simulink model "rear_differencial_dense_1"  (R2022b)
settings: Solver=FixedStepDiscrete  StartTime=0.0  StopTime=10.0  FixedStep=0.001  RelTol=1e-3  EnableMultiTasking=on
PreLoadFcn:
  | PowerOn_data
InitFcn:
  | EcoCoder_PreCheckLic();
values from neighbouring files (symbols this model uses):
  Accelerate_Percent_BreakPoints = uint8([0  2  5  10  20  30  40  50  60  70  80  90  100])    [PowerOn_data.m]
  MotorSpeed_BreakPoints = uint16(linspace(0,18000,13))    [PowerOn_data.m]
  Torque_Table = int8([ ... (first row only)    [PowerOn_data.m]
undefined symbols (not defined in the file or in its folder): HV_Botton, Inverter_Button, SC_Closed
libraries: CoderSF_BSW_Libs x83, SF_CanService_Libs x17, CoderSF_ADC2Volt_Libs x5, simulink x2, dspswit3 x1
(part 1 of 2)
settings Model: Param_HCUVersion=EV22297A  Creator=hxf  LastModifiedBy=Woler
settings SolverCC: AlgebraicLoopSolver=TrustRegion
settings DataIOCC: SaveFormat=Structure  SignalLoggingSaveFormat=ModelDataLogs  SaveOutput=off  SignalLogging=off  DSMLogging=off  SaveTime=off  ReturnWorkspaceOutputs=off
settings OptimizationCC: DefaultParameterBehavior=Inlined  InlineInvariantSignals=on  EnhancedBackFolding=on  StrengthReduction=on  EnableMemcpy=off  PassReuseOutputArgsAs=Individual arguments  EfficientFloat2IntCast=on  LifeSpan=1  SimCompilerOptimization=on  OptimizeBlockOrder=speed  DifferentSizesBufferReuse=on  EfficientTunableParamExpr=on
settings DebuggingCC: AlgebraicLoopMsg=none  ArtificialAlgebraicLoopMsg=none  SaveWithDisabledLinksMsg=none  SaveWithParameterizedLinksMsg=none  CheckSSInitialOutputMsg=off  UnderspecifiedInitializationDetection=Classic  SignalResolutionControl=TryResolveAll  BlockPriorityViolationMsg=error  MinStepSizeMsg=none  InheritedTsInSrcMsg=none  MultiTaskDSMMsg=none  MultiTaskCondExecSysMsg=none  MultiTaskRateTransMsg=warning  TasksWithSamePriorityMsg=none  SigSpecEnsureSampleTimeMsg=none  IntegerOverflowMsg=error  Int32ToFloatConvMsg=none  ParameterPrecisionLossMsg=none  ParameterTunabilityLossMsg=none  FixptConstOverflowMsg=error  FcnCallInpInsideContextMsg=warning  UnconnectedInputMsg=error  UnconnectedOutputMsg=error  UnconnectedLineMsg=error  FrameProcessingCompatibilityMsg=none  BusObjectLabelMismatch=none  RootOutportRequireBusObject=none  UnknownTsInhSupMsg=none  ModelReferenceDataLoggingMessage=none  OperatingPointInterfaceChecksumMismatchMsg=none  SFUnusedDataAndEventsDiag=none  SFUnexpectedBacktrackingDiag=none  SFInvalidInputDataAccessInChartInitDiag=none  SFNoUnconditionalDefaultTransitionDiag=none  SFTransitionOutsideNaturalParentDiag=none  SFUnreachableExecutionPathDiag=none  SFMachineParentedDataDiag=warning  ArithmeticOperatorsInVariantConditions=warning
settings HardwareCC: ProdBitPerPointer=32  ProdBitPerSizeT=32  ProdBitPerPtrDiffT=32  ProdLargestAtomicFloat=None  ProdWordSize=32  ProdHWDeviceType=Infineon->TriCore
settings ModelReferenceCC: UpdateModelReferenceTargets=Force  EnableRefExpFcnMdlSchedulingChecks=on  ModelReferenceNumInstancesAllowed=Single  PropagateSignalLabelsOutOfModel=off
settings SFSimCC: SFSimEcho=off  MATLABDynamicMemAlloc=off  CustomCodeUndefinedFunction=UseInterfaceOnly
settings RTWCC: Description=Ecotrons TC27x  SystemTargetFile=EcoCoderTC27x.tlc  GenerateMakefile=off  TemplateMakefile=ert_default_tmf  RTWVerbose=off  RetainRTWFile=on  RTWCompilerOptimization=on
settings CodeAppCC: IgnoreCustomStorageClasses=off  OperatorAnnotations=on  CustomSymbolStrGlobalVar=$N$M  CustomSymbolStrType=$N$M  CustomSymbolStrFcn=$N$M  CustomSymbolStrFcnArg=$N$M  CustomSymbolStrBlkIO=$N$M  CustomSymbolStrMacro=$N$M
settings STFCustomTargetCC: UtilityFuncGeneration=Shared location  MultiwordLength=256  IncludeMdlTerminateFcn=off  CombineOutputUpdateFcns=on  SuppressErrorStatus=on  ERTCustomFileBanners=on  SupportComplex=off  SupportContinuousTime=off  SupportNonInlinedSFcns=off  MATLABClassNameForMDSCustomization=Simulink.SoftwareTarget.ERTCustomization  SystemTargetFile=EcoCoderTC27x.tlc
settings ERTTargetCC: UtilityFuncGeneration=Shared location  ParMdlRefBuildCompliant=off  CompOptLevelCompliant=off  ConcurrentExecutionCompliant=off  IncludeMdlTerminateFcn=off  SuppressErrorStatus=on  SupportComplex=off  RemoveResetFunc=off  ModelStepFunctionPrototypeControlCompliant=off  CPPClassGenCompliant=off  UseToolchainInfoCompliant=off  GenerateASAP2=on  InlinedParameterPlacement=NonHierarchical  ERTCustomFileTemplate=MPC5644A_file_process.tlc  ERTFilePackagingFormat=Compact  PreserveIfCondition=on  ConvertIfToSwitch=off  PreserveExternInFcnDecls=off  SuppressUnreachableDefaultCases=off

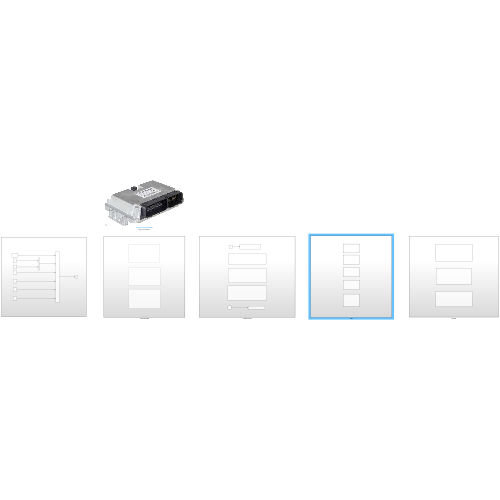
[thumbnail: Simulink's stored preview of the top-level diagram]
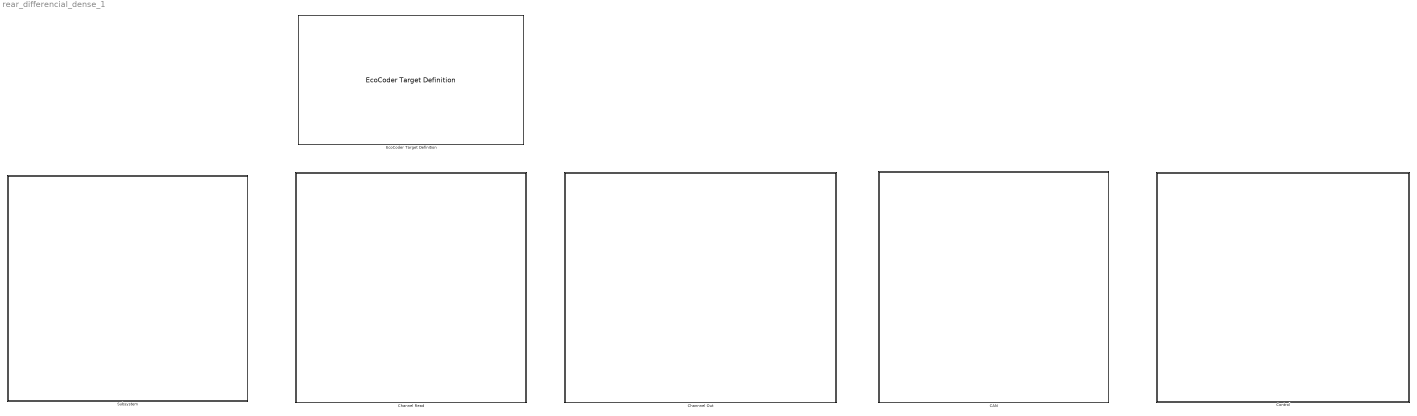
== system rear_differencial_dense_1 ==
  CAN : Subsystem
  Channel Read : Subsystem
  Channnel Out : Subsystem
  Control : Subsystem
  EcoCoder Target Definition : CoderSF_BSW_Libs/EcoCoder Target Definition  targetECU=EV22297A  EcoCoderBlockID=T001_Target  enNoTriggerCall=on  flgBlockReduction=on  flgShowDebugDisp=off  flgDisTargetOutFIleCounter=off  flgClearAllOldFiles=on  tc275_cal_len=hex2dec('00008000')  ipVal='192.168.0.123'  userName='nvidia'  passWord='nvidia'  workSpace='~/cmake_ws'  libraryLink=''  enExt=on  portExt=17725  internal_flash=[hex2dec('00020000'),hex2dec('000E0000')]  cal_rom_phy=[hex2dec('00010000'),hex2dec('00002000')]  cal_ram_wp=[hex2dec('4000F000'),hex2dec('00002000')]  cal_ram_msm=[hex2dec('40000000'),hex2dec('00002000')]  var_ram_wp=[hex2dec('40002000'),hex2dec('0000D000')]  write_back_fixed_ram=[hex2dec('40011000'),hex2dec('00001000')]  write_back_unfixed_ram=[hex2dec('40012000'),hex2dec('00001000')]  stack=[hex2dec('40013000'),hex2dec('00001000')]
      settings: AttributesFormatString=Target :%<targetECU>
  Subsystem : Subsystem

== system rear_differencial_dense_1/CAN ==
  CAN Definition : Subsystem
  CAN Read : Subsystem
  CAN Write : Subsystem
  Fixed CCP Slave Definition : CoderSF_BSW_Libs/CCP/Fixed CCP Slave Definition  ccp_enSet=on  ccp_disASW=off  channel=CAN_B  stationaddressSet=hex2dec('0112')  croidSet=hex2dec('200')  dtoidSet=hex2dec('201')  daqidSet=[hex2dec('210') hex2dec('211') hex2dec('212') hex2dec('213')]  daqpidSet=[hex2dec('0') hex2dec('0') hex2dec('0') hex2dec('0')]  daqlenSet=[hex2dec('A') hex2dec('20') hex2dec('30') hex2dec('50')]  daqperSet=[10 20 100 200]  EcoCoderBlockID=C002_CCP21Conf
  Write CAN Measurement : Subsystem

== system rear_differencial_dense_1/Channel Read ==
  ADC : Subsystem
  DI : Subsystem
  Multi_geer_knob : Subsystem

== system rear_differencial_dense_1/Channnel Out ==
  Constant : Constant  OutDataTypeStr=boolean
  Constant1 : Constant  OutDataTypeStr=boolean
  Power Control Output : CoderSF_BSW_Libs/System Management Blocks/Power Control Output  channel=PWR5V3
  Switch Output : CoderSF_BSW_Libs/Digital I//O/Switch Output  channel=HSO07
  水泵风扇 : Subsystem
  电池箱ACC_on : Subsystem
  蜂鸣器 : Subsystem
  wires:
  Constant1/1 -> Power Control Output/1
  Constant/1 -> Switch Output/1

== system rear_differencial_dense_1/Control ==
  Motor_Enable : Subsystem
  StateMachine : Subsystem
  Torque_Control : Subsystem

== system rear_differencial_dense_1/Subsystem ==
  Bus Creator : BusCreator  Inputs=Wheelbase,Distribution of Axle Load,Front Length,Rear Length,Front Track Width,Rear Track Width
  Divide : Product  Inputs=*/
  Front Length : Constant  Value=0.79
  Front Mass : Constant  Value=110
  Front Track Width : Constant  Value=1.2
  Rear Length : Constant  Value=0.79
  Rear Mass : Constant  Value=135
  Rear Track Width : Constant  Value=1.16
  Terminator : Terminator
  Wheelbase : Constant  Value=1.58
  wires:
  Front Mass/1 -> Divide/1
  Rear Mass/1 -> Divide/2
  Divide/1 -> Bus Creator/2  "Distribution of Axle Load"
  Wheelbase/1 -> Bus Creator/1  "Wheelbase"
  Front Length/1 -> Bus Creator/3  "Front Length"
  Rear Length/1 -> Bus Creator/4  "Rear Length"
  Front Track Width/1 -> Bus Creator/5  "Front Track Width"
  Rear Track Width/1 -> Bus Creator/6  "Rear Track Width"
  Bus Creator/1 -> Terminator/1

== system rear_differencial_dense_1/CAN/CAN Definition ==
  CAN Channel Definition : CoderSF_BSW_Libs/CAN/CAN Channel Definition  channel=CAN_A  can_en=on  can_idfilter=off  can_rxextended=off  can_rxMask=hex2dec('7ff')  can_rxID=hex2dec('100')  can_baudrateIndex=250  can_txbuffer_size=200  can_rxbuffer_size=1  can_en_fd=off  nominalSamplePoint=7500  can_baudrateIndex_data=500  fastSamplePoint=7500  canfd_txbuffer_size=5  EcoCoderBlockID=C001_CANDef
  CAN Channel Definition1 : CoderSF_BSW_Libs/CAN/CAN Channel Definition  channel=CAN_B  can_en=on  can_idfilter=off  can_rxextended=off  can_rxMask=hex2dec('7ff')  can_rxID=hex2dec('100')  can_baudrateIndex=500  can_txbuffer_size=200  can_rxbuffer_size=1  can_en_fd=off  nominalSamplePoint=7500  can_baudrateIndex_data=500  fastSamplePoint=7500  canfd_txbuffer_size=5  EcoCoderBlockID=C001_CANDef
  CAN Channel Definition2 : CoderSF_BSW_Libs/CAN/CAN Channel Definition  channel=CAN_C  can_en=on  can_idfilter=off  can_rxextended=off  can_rxMask=hex2dec('7ff')  can_rxID=hex2dec('100')  can_baudrateIndex=500  can_txbuffer_size=20  can_rxbuffer_size=1  can_en_fd=off  nominalSamplePoint=7500  can_baudrateIndex_data=500  fastSamplePoint=7500  canfd_txbuffer_size=5  EcoCoderBlockID=C001_CANDef
  CAN Channel Definition3 : CoderSF_BSW_Libs/CAN/CAN Channel Definition  channel=CAN_D  can_en=on  can_idfilter=off  can_rxextended=off  can_rxMask=hex2dec('7ff')  can_rxID=hex2dec('100')  can_baudrateIndex=500  can_txbuffer_size=20  can_rxbuffer_size=1  can_en_fd=off  nominalSamplePoint=7500  can_baudrateIndex_data=500  fastSamplePoint=7500  canfd_txbuffer_size=5  EcoCoderBlockID=C001_CANDef
  CAN Channel Definition4 : CoderSF_BSW_Libs/CAN/CAN Channel Definition  channel=CAN_E  can_en=on  can_idfilter=off  can_rxextended=off  can_rxMask=hex2dec('7ff')  can_rxID=hex2dec('100')  can_baudrateIndex=250  can_txbuffer_size=20  can_rxbuffer_size=1  can_en_fd=off  nominalSamplePoint=7500  can_baudrateIndex_data=500  fastSamplePoint=7500  canfd_txbuffer_size=5  EcoCoderBlockID=C001_CANDef

== system rear_differencial_dense_1/CAN/CAN Read ==
  BMS_CAN : Subsystem
  Motor_CAN : Subsystem
  SAS__CAN : Subsystem

== system rear_differencial_dense_1/CAN/CAN Write ==
  Send_To_Inverter : Subsystem
  Send_To_Recorder : Subsystem

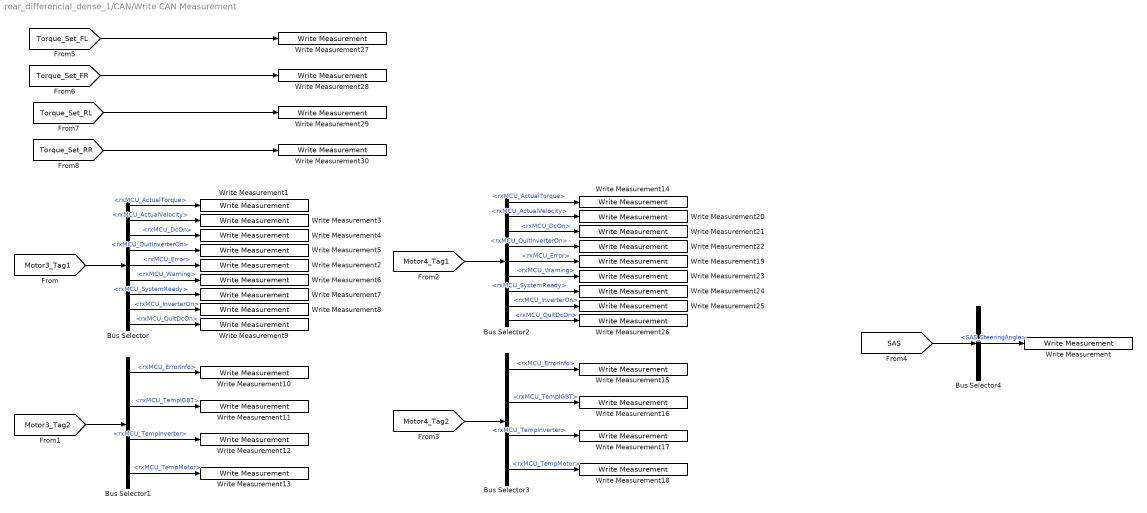
== system rear_differencial_dense_1/CAN/Write CAN Measurement ==
  Bus Selector : BusSelector  OutputSignals=rxMCU_ActualTorque,rxMCU_ActualVelocity,rxMCU_DcOn,rxMCU_QuitInverterOn,rxMCU_Error,rxMCU_Warning,rxMCU_SystemReady,rxMCU_InverterOn,rxMCU_QuitDcOn
  Bus Selector1 : BusSelector  OutputSignals=rxMCU_ErrorInfo,rxMCU_TempIGBT,rxMCU_TempInverter,rxMCU_TempMotor
  Bus Selector2 : BusSelector  OutputSignals=rxMCU_ActualTorque,rxMCU_ActualVelocity,rxMCU_DcOn,rxMCU_QuitInverterOn,rxMCU_Error,rxMCU_Warning,rxMCU_SystemReady,rxMCU_InverterOn,rxMCU_QuitDcOn
  Bus Selector3 : BusSelector  OutputSignals=rxMCU_ErrorInfo,rxMCU_TempIGBT,rxMCU_TempInverter,rxMCU_TempMotor
  Bus Selector4 : BusSelector  OutputSignals=SAS_SteeringAngle
  Write Measurement : CoderSF_BSW_Libs/Calibration & Measurement/Write Measurement  variable_name=Steering_Angle  variable_value=0  variable_type=single  numD=1  unitStr=""  descStr=""
      settings: AttributesFormatString=type:%<variable_type> Dimensions:%<numD>
  Write Measurement1 : CoderSF_BSW_Libs/Calibration & Measurement/Write Measurement  variable_name=RL_Actual_Torque  variable_value=0  variable_type=single  numD=1  unitStr=""  descStr=""
      settings: AttributesFormatString=type:%<variable_type> Dimensions:%<numD>
  Write Measurement10 : CoderSF_BSW_Libs/Calibration & Measurement/Write Measurement  variable_name=RL_Error_Info  variable_value=0  variable_type=uint16  numD=1  unitStr=""  descStr=""
      settings: AttributesFormatString=type:%<variable_type> Dimensions:%<numD>
  Write Measurement11 : CoderSF_BSW_Libs/Calibration & Measurement/Write Measurement  variable_name=RL_TempIGBT  variable_value=0  variable_type=single  numD=1  unitStr=""  descStr=""
      settings: AttributesFormatString=type:%<variable_type> Dimensions:%<numD>
  Write Measurement12 : CoderSF_BSW_Libs/Calibration & Measurement/Write Measurement  variable_name=RL_TempInverter  variable_value=0  variable_type=single  numD=1  unitStr=""  descStr=""
      settings: AttributesFormatString=type:%<variable_type> Dimensions:%<numD>
  Write Measurement13 : CoderSF_BSW_Libs/Calibration & Measurement/Write Measurement  variable_name=RL_TempMotor  variable_value=0  variable_type=single  numD=1  unitStr=""  descStr=""
      settings: AttributesFormatString=type:%<variable_type> Dimensions:%<numD>
  Write Measurement14 : CoderSF_BSW_Libs/Calibration & Measurement/Write Measurement  variable_name=RR_Actual_Torque  variable_value=0  variable_type=single  numD=1  unitStr=""  descStr=""
      settings: AttributesFormatString=type:%<variable_type> Dimensions:%<numD>
  Write Measurement15 : CoderSF_BSW_Libs/Calibration & Measurement/Write Measurement  variable_name=RR_Error_Info  variable_value=0  variable_type=uint16  numD=1  unitStr=""  descStr=""
      settings: AttributesFormatString=type:%<variable_type> Dimensions:%<numD>
  Write Measurement16 : CoderSF_BSW_Libs/Calibration & Measurement/Write Measurement  variable_name=RR_TempIGBT  variable_value=0  variable_type=single  numD=1  unitStr=""  descStr=""
      settings: AttributesFormatString=type:%<variable_type> Dimensions:%<numD>
  Write Measurement17 : CoderSF_BSW_Libs/Calibration & Measurement/Write Measurement  variable_name=RR_TempInverter  variable_value=0  variable_type=single  numD=1  unitStr=""  descStr=""
      settings: AttributesFormatString=type:%<variable_type> Dimensions:%<numD>
  Write Measurement18 : CoderSF_BSW_Libs/Calibration & Measurement/Write Measurement  variable_name=RR_TempMotor  variable_value=0  variable_type=single  numD=1  unitStr=""  descStr=""
      settings: AttributesFormatString=type:%<variable_type> Dimensions:%<numD>
  Write Measurement19 : CoderSF_BSW_Libs/Calibration & Measurement/Write Measurement  variable_name=RR_Error  variable_value=0  variable_type=boolean  numD=1  unitStr=""  descStr=""
      settings: AttributesFormatString=type:%<variable_type> Dimensions:%<numD>
  Write Measurement2 : CoderSF_BSW_Libs/Calibration & Measurement/Write Measurement  variable_name=RL_Error  variable_value=0  variable_type=boolean  numD=1  unitStr=""  descStr=""
      settings: AttributesFormatString=type:%<variable_type> Dimensions:%<numD>
  Write Measurement20 : CoderSF_BSW_Libs/Calibration & Measurement/Write Measurement  variable_name=RR_Actual_Velocity  variable_value=0  variable_type=int16  numD=1  unitStr=""  descStr=""
      settings: AttributesFormatString=type:%<variable_type> Dimensions:%<numD>
  Write Measurement21 : CoderSF_BSW_Libs/Calibration & Measurement/Write Measurement  variable_name=RR_DCon  variable_value=0  variable_type=boolean  numD=1  unitStr=""  descStr=""
      settings: AttributesFormatString=type:%<variable_type> Dimensions:%<numD>
  Write Measurement22 : CoderSF_BSW_Libs/Calibration & Measurement/Write Measurement  variable_name=RR_Quit_Inverter_on  variable_value=0  variable_type=boolean  numD=1  unitStr=""  descStr=""
      settings: AttributesFormatString=type:%<variable_type> Dimensions:%<numD>
  Write Measurement23 : CoderSF_BSW_Libs/Calibration & Measurement/Write Measurement  variable_name=RR_Warning  variable_value=0  variable_type=boolean  numD=1  unitStr=""  descStr=""
      settings: AttributesFormatString=type:%<variable_type> Dimensions:%<numD>
  Write Measurement24 : CoderSF_BSW_Libs/Calibration & Measurement/Write Measurement  variable_name=RR_System_Ready  variable_value=0  variable_type=boolean  numD=1  unitStr=""  descStr=""
      settings: AttributesFormatString=type:%<variable_type> Dimensions:%<numD>
  Write Measurement25 : CoderSF_BSW_Libs/Calibration & Measurement/Write Measurement  variable_name=RR_Inverter_on  variable_value=0  variable_type=boolean  numD=1  unitStr=""  descStr=""
      settings: AttributesFormatString=type:%<variable_type> Dimensions:%<numD>
  Write Measurement26 : CoderSF_BSW_Libs/Calibration & Measurement/Write Measurement  variable_name=RR_QuitDCon  variable_value=0  variable_type=boolean  numD=1  unitStr=""  descStr=""
      settings: AttributesFormatString=type:%<variable_type> Dimensions:%<numD>
  Write Measurement27 : CoderSF_BSW_Libs/Calibration & Measurement/Write Measurement  variable_name=Torque_Set_FL  variable_value=0  variable_type=uint16  numD=1  unitStr=""  descStr=""
      settings: AttributesFormatString=type:%<variable_type> Dimensions:%<numD>
  Write Measurement28 : CoderSF_BSW_Libs/Calibration & Measurement/Write Measurement  variable_name=Torque_Set_FR  variable_value=0  variable_type=uint16  numD=1  unitStr=""  descStr=""
      settings: AttributesFormatString=type:%<variable_type> Dimensions:%<numD>
  Write Measurement29 : CoderSF_BSW_Libs/Calibration & Measurement/Write Measurement  variable_name=Torque_Set_RL  variable_value=0  variable_type=uint16  numD=1  unitStr=""  descStr=""
      settings: AttributesFormatString=type:%<variable_type> Dimensions:%<numD>
  Write Measurement3 : CoderSF_BSW_Libs/Calibration & Measurement/Write Measurement  variable_name=RL_Actual_Velocity  variable_value=0  variable_type=int16  numD=1  unitStr=""  descStr=""
      settings: AttributesFormatString=type:%<variable_type> Dimensions:%<numD>
  Write Measurement30 : CoderSF_BSW_Libs/Calibration & Measurement/Write Measurement  variable_name=Torque_Set_RR  variable_value=0  variable_type=uint16  numD=1  unitStr=""  descStr=""
      settings: AttributesFormatString=type:%<variable_type> Dimensions:%<numD>
  Write Measurement4 : CoderSF_BSW_Libs/Calibration & Measurement/Write Measurement  variable_name=RL_DCon  variable_value=0  variable_type=boolean  numD=1  unitStr=""  descStr=""
      settings: AttributesFormatString=type:%<variable_type> Dimensions:%<numD>
  Write Measurement5 : CoderSF_BSW_Libs/Calibration & Measurement/Write Measurement  variable_name=RL_Quit_Inverter_on  variable_value=0  variable_type=boolean  numD=1  unitStr=""  descStr=""
      settings: AttributesFormatString=type:%<variable_type> Dimensions:%<numD>
  Write Measurement6 : CoderSF_BSW_Libs/Calibration & Measurement/Write Measurement  variable_name=RL_Warning  variable_value=0  variable_type=boolean  numD=1  unitStr=""  descStr=""
      settings: AttributesFormatString=type:%<variable_type> Dimensions:%<numD>
  Write Measurement7 : CoderSF_BSW_Libs/Calibration & Measurement/Write Measurement  variable_name=RL_System_Ready  variable_value=0  variable_type=boolean  numD=1  unitStr=""  descStr=""
      settings: AttributesFormatString=type:%<variable_type> Dimensions:%<numD>
  Write Measurement8 : CoderSF_BSW_Libs/Calibration & Measurement/Write Measurement  variable_name=RL_Inverter_on  variable_value=0  variable_type=boolean  numD=1  unitStr=""  descStr=""
      settings: AttributesFormatString=type:%<variable_type> Dimensions:%<numD>
  Write Measurement9 : CoderSF_BSW_Libs/Calibration & Measurement/Write Measurement  variable_name=RL_QuitDCon  variable_value=0  variable_type=boolean  numD=1  unitStr=""  descStr=""
      settings: AttributesFormatString=type:%<variable_type> Dimensions:%<numD>
  wires:
  Bus Selector1/4 -> Write Measurement13/1  "<rxMCU_TempMotor>"
  Bus Selector/1 -> Write Measurement1/1  "<rxMCU_ActualTorque>"
  Bus Selector2/9 -> Write Measurement26/1  "<rxMCU_QuitDcOn>"
  Bus Selector/2 -> Write Measurement3/1  "<rxMCU_ActualVelocity>"
  Bus Selector2/6 -> Write Measurement23/1  "<rxMCU_Warning>"
  Bus Selector/9 -> Write Measurement9/1  "<rxMCU_QuitDcOn>"
  Bus Selector/4 -> Write Measurement5/1  "<rxMCU_QuitInverterOn>"
  Bus Selector3/1 -> Write Measurement15/1  "<rxMCU_ErrorInfo>"
  Bus Selector3/3 -> Write Measurement17/1  "<rxMCU_TempInverter>"
  Bus Selector/3 -> Write Measurement4/1  "<rxMCU_DcOn>"
  [Motor3_Tag2] -> Bus Selector1/1
  Bus Selector/6 -> Write Measurement6/1  "<rxMCU_Warning>"
  Bus Selector/8 -> Write Measurement8/1  "<rxMCU_InverterOn>"
  Bus Selector/5 -> Write Measurement2/1  "<rxMCU_Error>"
  [Motor4_Tag2] -> Bus Selector3/1
  [Motor3_Tag1] -> Bus Selector/1
  Bus Selector2/2 -> Write Measurement20/1  "<rxMCU_ActualVelocity>"
  Bus Selector2/1 -> Write Measurement14/1  "<rxMCU_ActualTorque>"
  Bus Selector3/4 -> Write Measurement18/1  "<rxMCU_TempMotor>"
  Bus Selector2/5 -> Write Measurement19/1  "<rxMCU_Error>"
  Bus Selector2/8 -> Write Measurement25/1  "<rxMCU_InverterOn>"
  Bus Selector3/2 -> Write Measurement16/1  "<rxMCU_TempIGBT>"
  Bus Selector1/3 -> Write Measurement12/1  "<rxMCU_TempInverter>"
  [Motor4_Tag1] -> Bus Selector2/1
  Bus Selector2/4 -> Write Measurement22/1  "<rxMCU_QuitInverterOn>"
  Bus Selector2/7 -> Write Measurement24/1  "<rxMCU_SystemReady>"
  Bus Selector2/3 -> Write Measurement21/1  "<rxMCU_DcOn>"
  Bus Selector1/2 -> Write Measurement11/1  "<rxMCU_TempIGBT>"
  Bus Selector1/1 -> Write Measurement10/1  "<rxMCU_ErrorInfo>"
  Bus Selector/7 -> Write Measurement7/1  "<rxMCU_SystemReady>"
  [SAS] -> Bus Selector4/1
  Bus Selector4/1 -> Write Measurement/1  "<SAS_SteeringAngle>"
  [Torque_Set_RR] -> Write Measurement30/1
  [Torque_Set_RL] -> Write Measurement29/1
  [Torque_Set_FR] -> Write Measurement28/1
  [Torque_Set_FL] -> Write Measurement27/1

== system rear_differencial_dense_1/Channel Read/ADC ==
  "ADC Reading " : Subsystem
  Bus Creator : BusCreator  Inputs=4
  Terminator : Terminator
  tag scope: Accelerate_Percent=global, Accelerate_Unreliable=global, Brake_Percent=global, LV_Batterry_Voltage=global
  wires:
  [Brake_Percent] -> Bus Creator/3
  "ADC Reading "/1(Accelerate_Unreliable) -> [Accelerate_Unreliable]
  [Accelerate_Percent] -> Bus Creator/2
  [Accelerate_Unreliable] -> Bus Creator/1
  "ADC Reading "/3(Brake_percent) -> [Brake_Percent]
  Bus Creator/1 -> Terminator/1
  "ADC Reading "/2(Accelerate_Percent) -> [Accelerate_Percent]
  [LV_Batterry_Voltage] -> Bus Creator/4
  "ADC Reading "/4(LV_battery_voltage) -> [LV_Batterry_Voltage]

== system rear_differencial_dense_1/Channel Read/DI ==
  Bus Creator : BusCreator  Inputs=HV_Botton,Inverter_Button,SC_Closed
  Switch Input : CoderSF_BSW_Libs/Digital I//O/Switch Input  portNum=DI01
  Switch Input1 : CoderSF_BSW_Libs/Digital I//O/Switch Input  portNum=DI03
  Switch Input2 : CoderSF_BSW_Libs/Digital I//O/Switch Input  portNum=DI02
  Write Measurement : CoderSF_BSW_Libs/Calibration & Measurement/Write Measurement  variable_name=SC_Closed  variable_value=0  variable_type=boolean  numD=1  unitStr=""  descStr=""
      settings: AttributesFormatString=type:%<variable_type> Dimensions:%<numD>
  tag scope: DI=global
  wires:
  Bus Creator/1 -> [DI]
  Switch Input/1 -> Bus Creator/1  "HV_Botton"
  Switch Input1/1 -> Bus Creator/3, Write Measurement/1  "SC_Closed"
  Switch Input2/1 -> Bus Creator/2  "Inverter_Button"

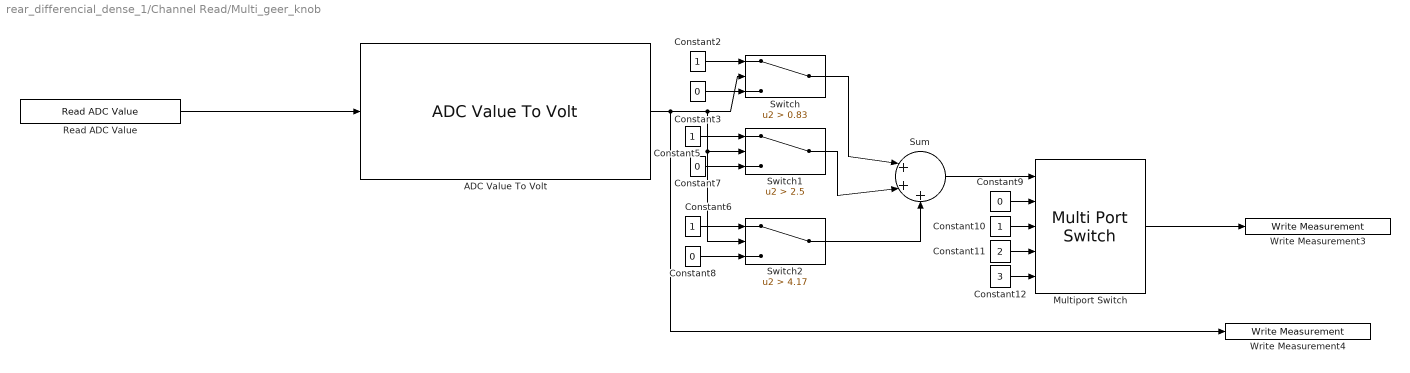
== system rear_differencial_dense_1/Channel Read/Multi_geer_knob ==
  ADC Value To Volt : CoderSF_ADC2Volt_Libs/ADC Value To Volt  ResValue=12  RefValue=5  TypeOut=single  WithDiv=off  DivValue=16  SerValue=100
  Constant10 : Constant  OutDataTypeStr=uint16
  Constant11 : Constant  Value=2  OutDataTypeStr=uint16
  Constant12 : Constant  Value=3  OutDataTypeStr=uint16
  Constant2 : Constant  OutDataTypeStr=single
  Constant3 : Constant  Value=0  OutDataTypeStr=single
  Constant5 : Constant  OutDataTypeStr=uint16
  Constant6 : Constant  OutDataTypeStr=uint16
  Constant7 : Constant  Value=0  OutDataTypeStr=uint16
  Constant8 : Constant  Value=0  OutDataTypeStr=uint16
  Constant9 : Constant  Value=0  OutDataTypeStr=uint16
  Multiport Switch : MultiPortSwitch  DataPortOrder=Zero-based contiguous  Inputs=4  zeroidx=on  SaturateOnIntegerOverflow=off  InputSameDT=off
  Read ADC Value : CoderSF_BSW_Libs/ADC/Read ADC Value  channel=4
  Sum : Sum  Inputs=|+++  AccumDataTypeStr=uint16
  Switch : Switch  Criteria=u2 > Threshold  Threshold=0.83  OutDataTypeStr=uint16  SaturateOnIntegerOverflow=off  InputSameDT=off
  Switch1 : Switch  Criteria=u2 > Threshold  Threshold=2.5  OutDataTypeStr=uint16  SaturateOnIntegerOverflow=off  InputSameDT=off
  Switch2 : Switch  Criteria=u2 > Threshold  Threshold=4.17  OutDataTypeStr=uint16  SaturateOnIntegerOverflow=off  InputSameDT=off
  Write Measurement3 : CoderSF_BSW_Libs/Calibration & Measurement/Write Measurement  variable_name=Multi_gear_knob  variable_value=0  variable_type=uint16  numD=1  unitStr=""  descStr=""
      settings: AttributesFormatString=type:%<variable_type> Dimensions:%<numD>
  Write Measurement4 : CoderSF_BSW_Libs/Calibration & Measurement/Write Measurement  variable_name=KNOB_VOLTAGE  variable_value=0  variable_type=single  numD=1  unitStr=""  descStr=""
      settings: AttributesFormatString=type:%<variable_type> Dimensions:%<numD>
  wires:
  Sum/1 -> Multiport Switch/1
  Multiport Switch/1 -> Write Measurement3/1
  Constant2/1 -> Switch/1
  Constant3/1 -> Switch/3
  Constant12/1 -> Multiport Switch/5
  Constant6/1 -> Switch2/1
  Constant9/1 -> Multiport Switch/2
  Switch1/1 -> Sum/2
  Constant11/1 -> Multiport Switch/4
  Switch/1 -> Sum/1
  Constant7/1 -> Switch1/3
  Constant5/1 -> Switch1/1
  Switch2/1 -> Sum/3
  ADC Value To Volt/1 -> Write Measurement4/1, Switch2/2, Switch1/2, Switch/2
  Constant8/1 -> Switch2/3
  Read ADC Value/1 -> ADC Value To Volt/1
  Constant10/1 -> Multiport Switch/3

== system rear_differencial_dense_1/Channnel Out/水泵风扇 ==
  Compare To Constant : simulink/Logic and Bit Operations/Compare To Constant  relop===  const=1  OutDataTypeStr=boolean
  水泵风扇1 : CoderSF_BSW_Libs/Digital I//O/Switch Output  channel=HSO01
  水泵风扇2 : CoderSF_BSW_Libs/Digital I//O/Switch Output  channel=HSO02
  wires:
  [Invertor_Enable] -> Compare To Constant/1
  Compare To Constant/1 -> 水泵风扇1/1, 水泵风扇2/1

== system rear_differencial_dense_1/Channnel Out/电池箱ACC_on ==
  Constant2 : Constant  OutDataTypeStr=boolean
  电池箱 ACC_on : CoderSF_BSW_Libs/Digital I//O/Switch Output  channel=HSO05
  wires:
  Constant2/1 -> 电池箱 ACC_on/1

== system rear_differencial_dense_1/Channnel Out/蜂鸣器 ==
  AND1 : Logic  IconShape=distinctive  AllPortsSameDT=off  OutDataTypeStr=boolean
  Constant : Constant  Value=0  OutDataTypeStr=boolean
  Constant1 : Constant  OutDataTypeStr=boolean
  Counter : dspswit3/Counter  Direction=Up  CountEvent=Non-zero sample  CounterSize=32 bits  MaxCount=255  InitialCount=0  Output=Count  HitValue=30  ResetInput=on  SamplesPerFrame=1  Ts=1  CntDtype=uint32  HitDtype=Boolean
  NOT2 : Logic  Operator=NOT  IconShape=distinctive  AllPortsSameDT=off  OutDataTypeStr=boolean
  Switch : Switch  Criteria=u2 > Threshold  Threshold=2000  OutDataTypeStr=boolean  SaturateOnIntegerOverflow=off  InputSameDT=off
  蜂鸣器 : CoderSF_BSW_Libs/Digital I//O/Switch Output  channel=HSO08
  wires:
  [Invertor_Enable] -> NOT2/1, AND1/1, Counter/1
  Constant1/1 -> Switch/3
  Constant/1 -> Switch/1
  Counter/1 -> Switch/2
  NOT2/1 -> Counter/2
  Switch/1 -> AND1/2
  AND1/1 -> 蜂鸣器/1

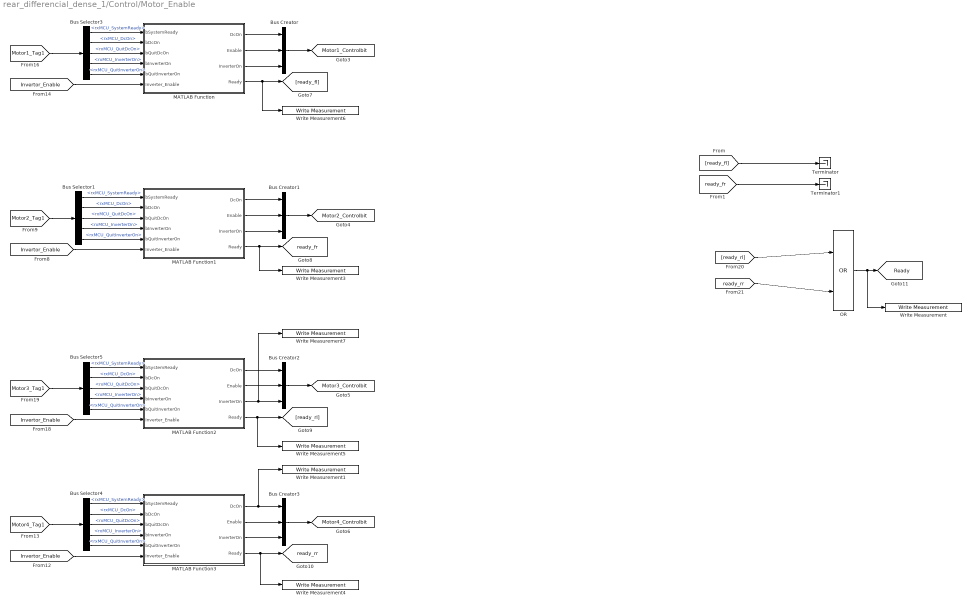
== system rear_differencial_dense_1/Control/Motor_Enable ==
  Bus Creator{,1..3} (4 alike) : BusCreator  Inputs=3
  Bus Selector{1,3..5} (4 alike) : BusSelector  OutputSignals=rxMCU_SystemReady,rxMCU_DcOn,rxMCU_QuitDcOn,rxMCU_InverterOn,rxMCU_QuitInverterOn
  MATLAB Function : MATLAB Function  TreatAsAtomicUnit=on
  MATLAB Function1 : MATLAB Function  TreatAsAtomicUnit=on
  MATLAB Function2 : MATLAB Function  TreatAsAtomicUnit=on
  MATLAB Function3 : MATLAB Function  TreatAsAtomicUnit=on
  OR : Logic  Operator=OR  IconShape=distinctive  AllPortsSameDT=off  OutDataTypeStr=boolean
  Terminator : Terminator
  Terminator1 : Terminator
  Write Measurement : CoderSF_BSW_Libs/Calibration & Measurement/Write Measurement  variable_name=Ready  variable_value=0  variable_type=boolean  numD=1  unitStr=""  descStr=""
      settings: AttributesFormatString=type:%<variable_type> Dimensions:%<numD>
  Write Measurement1 : CoderSF_BSW_Libs/Calibration & Measurement/Write Measurement  variable_name=InverterOn_State_RR  variable_value=0  variable_type=int16  numD=1  unitStr=""  descStr=""
      settings: AttributesFormatString=type:%<variable_type> Dimensions:%<numD>
  Write Measurement3 : CoderSF_BSW_Libs/Calibration & Measurement/Write Measurement  variable_name=ready_fr  variable_value=0  variable_type=int16  numD=1  unitStr=""  descStr=""
      settings: AttributesFormatString=type:%<variable_type> Dimensions:%<numD>
  Write Measurement4 : CoderSF_BSW_Libs/Calibration & Measurement/Write Measurement  variable_name=ready_rr  variable_value=0  variable_type=int16  numD=1  unitStr=""  descStr=""
      settings: AttributesFormatString=type:%<variable_type> Dimensions:%<numD>
  Write Measurement5 : CoderSF_BSW_Libs/Calibration & Measurement/Write Measurement  variable_name=ready_rl  variable_value=0  variable_type=int16  numD=1  unitStr=""  descStr=""
      settings: AttributesFormatString=type:%<variable_type> Dimensions:%<numD>
  Write Measurement6 : CoderSF_BSW_Libs/Calibration & Measurement/Write Measurement  variable_name=ready_fl  variable_value=0  variable_type=int16  numD=1  unitStr=""  descStr=""
      settings: AttributesFormatString=type:%<variable_type> Dimensions:%<numD>
  Write Measurement7 : CoderSF_BSW_Libs/Calibration & Measurement/Write Measurement  variable_name=InverterOn_State_RL  variable_value=0  variable_type=int16  numD=1  unitStr=""  descStr=""
      settings: AttributesFormatString=type:%<variable_type> Dimensions:%<numD>
  tag scope: Motor1_Controlbit=global, Motor2_Controlbit=global, Motor3_Controlbit=global, Motor4_Controlbit=global, Ready=global, ready_fr=global, ready_rr=global
  wires:
  MATLAB Function/2(Enable) -> Bus Creator/2
  [Invertor_Enable] -> MATLAB Function/6(Inverter_Enable)
  Bus Selector1/4 -> MATLAB Function1/4(bInverterOn)  "<rxMCU_InverterOn>"
  [Invertor_Enable] -> MATLAB Function2/6(Inverter_Enable)
  Bus Selector3/5 -> MATLAB Function/5(bQuitInverterOn)  "<rxMCU_QuitInverterOn>"
  Bus Selector4/4 -> MATLAB Function3/4(bInverterOn)  "<rxMCU_InverterOn>"
  MATLAB Function/3(InverterOn) -> Bus Creator/3
  MATLAB Function3/4(Ready) -> Write Measurement4/1, [ready_rr]
  OR/1 -> Write Measurement/1, [Ready]
  MATLAB Function/4(Ready) -> Write Measurement6/1, [ready_fl]
  Bus Selector3/2 -> MATLAB Function/2(bDcOn)  "<rxMCU_DcOn>"
  Bus Creator3/1 -> [Motor4_Controlbit]
  Bus Selector1/3 -> MATLAB Function1/3(bQuitDcOn)  "<rxMCU_QuitDcOn>"
  Bus Selector4/2 -> MATLAB Function3/2(bDcOn)  "<rxMCU_DcOn>"
  Bus Creator/1 -> [Motor1_Controlbit]
  Bus Selector4/1 -> MATLAB Function3/1(bSystemReady)  "<rxMCU_SystemReady>"
  Bus Selector1/2 -> MATLAB Function1/2(bDcOn)  "<rxMCU_DcOn>"
  MATLAB Function1/4(Ready) -> Write Measurement3/1, [ready_fr]
  [Invertor_Enable] -> MATLAB Function3/6(Inverter_Enable)
  Bus Selector5/3 -> MATLAB Function2/3(bQuitDcOn)  "<rxMCU_QuitDcOn>"
  MATLAB Function1/1(DcOn) -> Bus Creator1/1
  Bus Selector5/5 -> MATLAB Function2/5(bQuitInverterOn)  "<rxMCU_QuitInverterOn>"
  MATLAB Function3/3(InverterOn) -> Bus Creator3/3
  Bus Selector3/3 -> MATLAB Function/3(bQuitDcOn)  "<rxMCU_QuitDcOn>"
  MATLAB Function2/4(Ready) -> Write Measurement5/1, [ready_rl]
  MATLAB Function2/2(Enable) -> Bus Creator2/2
  MATLAB Function1/2(Enable) -> Bus Creator1/2
  [Motor4_Tag1] -> Bus Selector4/1
  Bus Selector3/4 -> MATLAB Function/4(bInverterOn)  "<rxMCU_InverterOn>"
  MATLAB Function/1(DcOn) -> Bus Creator/1
  Bus Selector5/2 -> MATLAB Function2/2(bDcOn)  "<rxMCU_DcOn>"
  Bus Selector3/1 -> MATLAB Function/1(bSystemReady)  "<rxMCU_SystemReady>"
  MATLAB Function1/3(InverterOn) -> Bus Creator1/3
  [Motor1_Tag1] -> Bus Selector3/1
  MATLAB Function2/1(DcOn) -> Bus Creator2/1
  [Invertor_Enable] -> MATLAB Function1/6(Inverter_Enable)
  MATLAB Function3/2(Enable) -> Bus Creator3/2
  Bus Selector5/4 -> MATLAB Function2/4(bInverterOn)  "<rxMCU_InverterOn>"
  MATLAB Function2/3(InverterOn) -> Write Measurement7/1, Bus Creator2/3
  Bus Selector4/5 -> MATLAB Function3/5(bQuitInverterOn)  "<rxMCU_QuitInverterOn>"
  [Motor3_Tag1] -> Bus Selector5/1
  Bus Selector5/1 -> MATLAB Function2/1(bSystemReady)  "<rxMCU_SystemReady>"
  Bus Selector1/1 -> MATLAB Function1/1(bSystemReady)  "<rxMCU_SystemReady>"
  Bus Selector1/5 -> MATLAB Function1/5(bQuitInverterOn)  "<rxMCU_QuitInverterOn>"
  [Motor2_Tag1] -> Bus Selector1/1
  Bus Creator2/1 -> [Motor3_Controlbit]
  Bus Creator1/1 -> [Motor2_Controlbit]
  Bus Selector4/3 -> MATLAB Function3/3(bQuitDcOn)  "<rxMCU_QuitDcOn>"
  [ready_rl] -> OR/1
  [ready_rr] -> OR/2
  [ready_fr] -> Terminator1/1
  [ready_fl] -> Terminator/1
  MATLAB Function3/1(DcOn) -> Write Measurement1/1, Bus Creator3/1

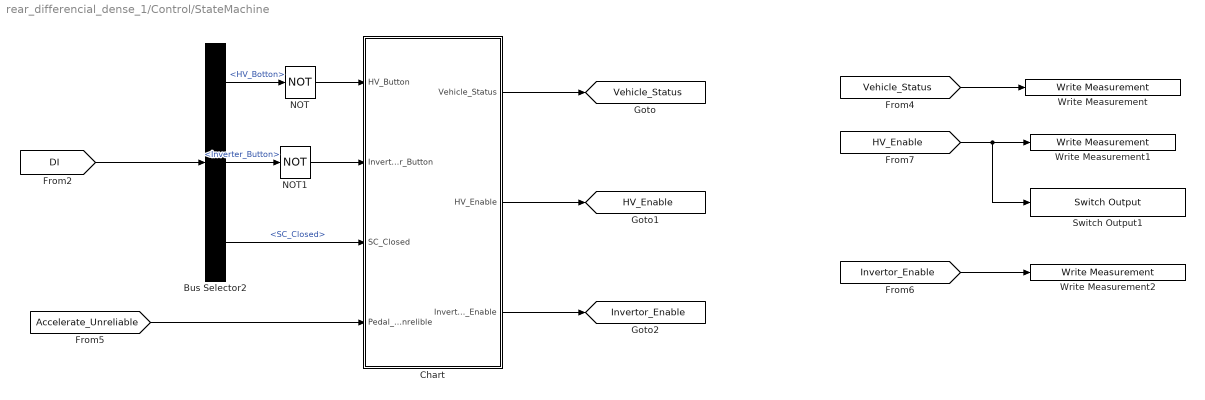
== system rear_differencial_dense_1/Control/StateMachine ==
  Bus Selector2 : BusSelector  OutputSignals=HV_Botton,Inverter_Button,SC_Closed
  Chart : Stateflow chart  TreatAsAtomicUnit=on
  NOT : Logic  Operator=NOT  IconShape=distinctive  AllPortsSameDT=off  OutDataTypeStr=boolean
  NOT1 : Logic  Operator=NOT  IconShape=distinctive  AllPortsSameDT=off  OutDataTypeStr=boolean
  Switch Output1 : CoderSF_BSW_Libs/Digital I//O/Switch Output  channel=HSO09
  Write Measurement : CoderSF_BSW_Libs/Calibration & Measurement/Write Measurement  variable_name=Vehicle_Status  variable_value=0  variable_type=single  numD=1  unitStr=""  descStr=""
      settings: AttributesFormatString=type:%<variable_type> Dimensions:%<numD>
  Write Measurement1 : CoderSF_BSW_Libs/Calibration & Measurement/Write Measurement  variable_name=HV_Enable  variable_value=0  variable_type=boolean  numD=1  unitStr=""  descStr=""
      settings: AttributesFormatString=type:%<variable_type> Dimensions:%<numD>
  Write Measurement2 : CoderSF_BSW_Libs/Calibration & Measurement/Write Measurement  variable_name=Invertor_Enable  variable_value=0  variable_type=boolean  numD=1  unitStr=""  descStr=""
      settings: AttributesFormatString=type:%<variable_type> Dimensions:%<numD>
  tag scope: HV_Enable=global, Invertor_Enable=global, Vehicle_Status=global
  wires:
  Bus Selector2/3 -> Chart/3(SC_Closed)  "<SC_Closed>"
  Chart/2(HV_Enable) -> [HV_Enable]
  Bus Selector2/1 -> NOT/1  "<HV_Botton>"
  Chart/1(Vehicle_Status) -> [Vehicle_Status]
  Chart/3(Invertor_Enable) -> [Invertor_Enable]
  [DI] -> Bus Selector2/1
  [Vehicle_Status] -> Write Measurement/1
  [Accelerate_Unreliable] -> Chart/4(Pedal_Unrelible)
  [Invertor_Enable] -> Write Measurement2/1
  [HV_Enable] -> Switch Output1/1, Write Measurement1/1
  NOT/1 -> Chart/1(HV_Button)
  Bus Selector2/2 -> NOT1/1  "<Inverter_Button>"
  NOT1/1 -> Chart/2(Invertor_Button)

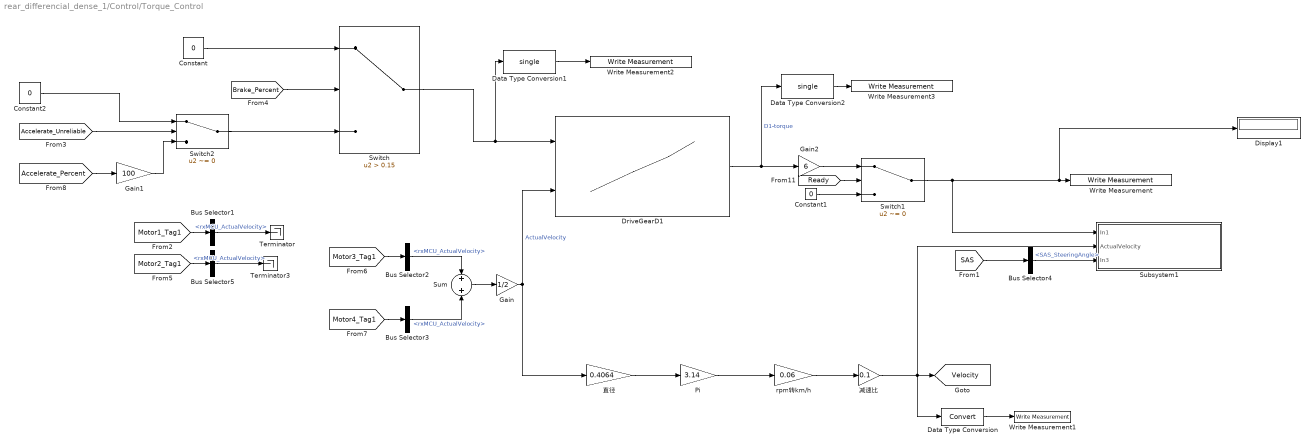
== system rear_differencial_dense_1/Control/Torque_Control ==
  Bus Selector{1..3,5} (4 alike) : BusSelector  OutputSignals=rxMCU_ActualVelocity
  Bus Selector4 : BusSelector  OutputSignals=SAS_SteeringAngle
  Constant : Constant  Value=0
  Constant1 : Constant  Value=0
  Constant2 : Constant  Value=0
  Data Type Conversion : DataTypeConversion  SaturateOnIntegerOverflow=off  RndMeth=Floor
  Data Type Conversion1 : DataTypeConversion  OutDataTypeStr=single  SaturateOnIntegerOverflow=off  RndMeth=Floor
  Data Type Conversion2 : DataTypeConversion  OutDataTypeStr=single  SaturateOnIntegerOverflow=off  RndMeth=Floor
  Display1 : Display
  DriveGearD1 : Lookup_n-D  BreakpointsForDimension1=Accelerate_Percent_BreakPoints  BreakpointsForDimension2=MotorSpeed_BreakPoints  BreakpointsForDimension1DataTypeStr=Inherit: Inherit from 'Breakpoint data'  BreakpointsForDimension2DataTypeStr=Inherit: Inherit from 'Breakpoint data'  IndexSearchMethod=Linear search  Table=Torque_Table  TableDataTypeStr=double  IntermediateResultsDataTypeStr=double  ExtrapMethod=Clip  InternalRulePriority=Speed  OutDataTypeStr=double  RndMeth=Simplest  FractionDataTypeStr=double  InputSameDT=off
      settings: InputPortMap=u0,u1
  Gain : Gain  Gain=1/2  ParamDataTypeStr=uint16  OutDataTypeStr=uint16
  Gain1 : Gain  Gain=100
  Gain2 : Gain  Gain=6
  Pi : Gain  Gain=3.14  OutDataTypeStr=single
  Subsystem1 : Subsystem
  Sum : Sum
  Switch : Switch  Criteria=u2 > Threshold  Threshold=0.15  SaturateOnIntegerOverflow=off  InputSameDT=off
  Switch1 : Switch  Criteria=u2 ~= 0  Threshold=0.1  OutDataTypeStr=int16  SaturateOnIntegerOverflow=off  InputSameDT=off
  Switch2 : Switch  Criteria=u2 ~= 0  SaturateOnIntegerOverflow=off  InputSameDT=off
  Terminator : Terminator
  Terminator3 : Terminator
  Write Measurement : CoderSF_BSW_Libs/Calibration & Measurement/Write Measurement  variable_name=torque_output  variable_value=0  variable_type=int16  numD=1  unitStr=""  descStr=""
      settings: AttributesFormatString=type:%<variable_type> Dimensions:%<numD>
  Write Measurement1 : CoderSF_BSW_Libs/Calibration & Measurement/Write Measurement  variable_name=actual_velocity  variable_value=0  variable_type=single  numD=1  unitStr=""  descStr=""
      settings: AttributesFormatString=type:%<variable_type> Dimensions:%<numD>
  Write Measurement2 : CoderSF_BSW_Libs/Calibration & Measurement/Write Measurement  variable_name=percent_raw  variable_value=0  variable_type=single  numD=1  unitStr=""  descStr=""
      settings: AttributesFormatString=type:%<variable_type> Dimensions:%<numD>
  Write Measurement3 : CoderSF_BSW_Libs/Calibration & Measurement/Write Measurement  variable_name=percent_out  variable_value=0  variable_type=single  numD=1  unitStr=""  descStr=""
      settings: AttributesFormatString=type:%<variable_type> Dimensions:%<numD>
  rpm转km/h : Gain  Gain=0.06  OutDataTypeStr=single
  减速比 : Gain  Gain=0.1  OutDataTypeStr=single
  直径 : Gain  Gain=0.4064  OutDataTypeStr=single
  tag scope: Velocity=global
  wires:
  Constant1/1 -> Switch1/3
  DriveGearD1/1 -> Data Type Conversion2/1, Gain2/1  "D1-torque"
  Gain2/1 -> Switch1/1
  Sum/1 -> Gain/1
  [Motor3_Tag1] -> Bus Selector2/1
  [Motor4_Tag1] -> Bus Selector3/1
  Gain/1 -> 直径/1, DriveGearD1/2  "ActualVelocity"
  Constant/1 -> Switch/1
  Switch/1 -> DriveGearD1/1, Data Type Conversion1/1
  Gain1/1 -> Switch2/3
  [Accelerate_Percent] -> Gain1/1
  [Accelerate_Unreliable] -> Switch2/2
  Constant2/1 -> Switch2/1
  Switch2/1 -> Switch/3
  [SAS] -> Bus Selector4/1
  [Brake_Percent] -> Switch/2
  直径/1 -> Pi/1
  Pi/1 -> rpm转km/h/1
  rpm转km/h/1 -> 减速比/1
  Bus Selector2/1 -> Sum/1  "<rxMCU_ActualVelocity>"
  Data Type Conversion/1 -> Write Measurement1/1
  减速比/1 -> Data Type Conversion/1, Subsystem1/2(ActualVelocity), [Velocity]
  Data Type Conversion1/1 -> Write Measurement2/1
  Data Type Conversion2/1 -> Write Measurement3/1
  Bus Selector5/1 -> Terminator3/1  "<rxMCU_ActualVelocity>"
  [Motor2_Tag1] -> Bus Selector5/1
  [Motor1_Tag1] -> Bus Selector1/1
  Bus Selector1/1 -> Terminator/1  "<rxMCU_ActualVelocity>"
  Bus Selector3/1 -> Sum/2  "<rxMCU_ActualVelocity>"
  Switch1/1 -> Subsystem1/1(In1), Display1/1, Write Measurement/1
  Bus Selector4/1 -> Subsystem1/3(In3)  "<SAS_SteeringAngle>"
  [Ready] -> Switch1/2

== system rear_differencial_dense_1/CAN/CAN Read/BMS_CAN ==
  Bus Creator : BusCreator  Inputs=9
  Bus Creator1 : BusCreator  Inputs=7
  Bus Creator2 : BusCreator  Inputs=9
  Read CAN Message : SF_CanService_Libs/Read CAN Message  typeCAN=Connected  channel=CAN_E  mEn=off  msgInfo=BCU_HCU_INFO_v3  msgItermStore=BMS_HCU_INFO  msgIterm=BMS_HCU_INFO  valid=on  stale=on  motoBit=off  setSignalName=on  flgCustomMonitorVariableRules=on  defineSignalName=off  prefixSignal=''  flgValTest=off  flgNoFixed=on  tSample=Task_Inherit  modeCode=Parameterless
  Read CAN Message1 : SF_CanService_Libs/Read CAN Message  typeCAN=Connected  channel=CAN_E  mEn=off  msgInfo=BCU_HCU_INFO_v3  msgItermStore=BMS_HCU_MAXV  msgIterm=BMS_HCU_MAXV  valid=on  stale=on  motoBit=off  setSignalName=on  flgCustomMonitorVariableRules=on  defineSignalName=off  prefixSignal=''  flgValTest=off  flgNoFixed=on  tSample=Task_Inherit  modeCode=Parameterless
  Read CAN Message2 : SF_CanService_Libs/Read CAN Message  typeCAN=Connected  channel=CAN_E  mEn=off  msgInfo=BCU_HCU_INFO_v3  msgItermStore=BMS_HCU_MAXT  msgIterm=BMS_HCU_MAXT  valid=on  stale=on  motoBit=off  setSignalName=on  flgCustomMonitorVariableRules=on  defineSignalName=off  prefixSignal=''  flgValTest=off  flgNoFixed=on  tSample=Task_Inherit  modeCode=Parameterless
  tag scope: BMS_INFO=global, BMS_MAXT=global, BMS_MAXV=global
  wires:
  Bus Creator/1 -> [BMS_INFO]
  Read CAN Message/3 -> Bus Creator/3  "BatVoltage"
  Read CAN Message/6 -> Bus Creator/6  "BatSoc"
  Read CAN Message/1 -> Bus Creator/1
  Read CAN Message/5 -> Bus Creator/5  "BatSoh"
  Read CAN Message/2 -> Bus Creator/2
  Read CAN Message/4 -> Bus Creator/4  "BatState"
  Read CAN Message/9 -> Bus Creator/9  "BatAlmLv"
  Read CAN Message/7 -> Bus Creator/7  "BatLife"
  Read CAN Message/8 -> Bus Creator/8  "BatCurrent"
  Read CAN Message1/1 -> Bus Creator1/1
  Read CAN Message1/2 -> Bus Creator1/2
  Read CAN Message1/3 -> Bus Creator1/3  "Unused_2"
  Read CAN Message1/4 -> Bus Creator1/4  "MinCellVoltNo"
  Read CAN Message1/5 -> Bus Creator1/5  "MaxCellVoltNo"
  Read CAN Message1/6 -> Bus Creator1/6  "MinCellVolt"
  Bus Creator1/1 -> [BMS_MAXV]
  Read CAN Message2/6 -> Bus Creator2/6  "MinTempNo"
  Read CAN Message2/1 -> Bus Creator2/1
  Read CAN Message2/4 -> Bus Creator2/4  "Heating_Ctl"
  Read CAN Message2/5 -> Bus Creator2/5  "Cooling_Ctl"
  Read CAN Message2/3 -> Bus Creator2/3  "Unused_1"
  Read CAN Message2/2 -> Bus Creator2/2
  Bus Creator2/1 -> [BMS_MAXT]
  Read CAN Message1/7 -> Bus Creator1/7  "MaxCellVolt"
  Read CAN Message2/7 -> Bus Creator2/7  "MaxTempNo"
  Read CAN Message2/8 -> Bus Creator2/8  "MinTemp"
  Read CAN Message2/9 -> Bus Creator2/9  "MaxTemp"

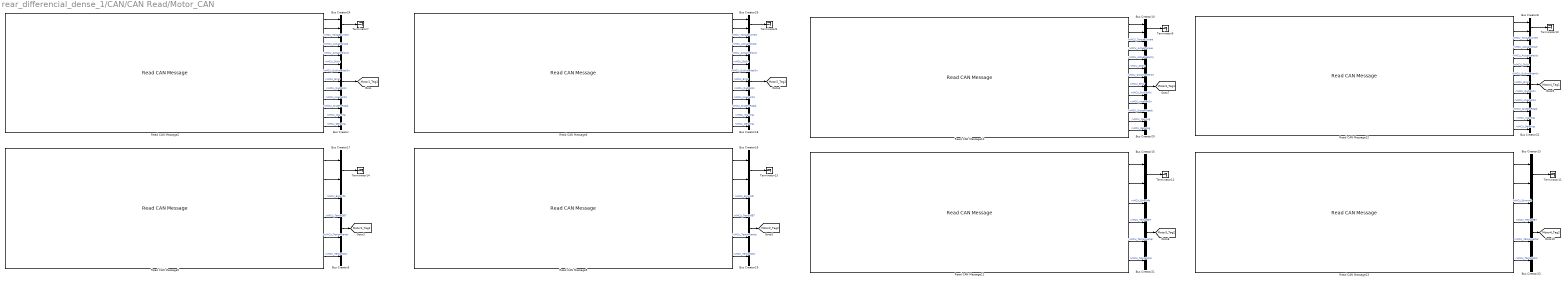
== system rear_differencial_dense_1/CAN/CAN Read/Motor_CAN ==
  Bus Creator{,18,20,22} (4 alike) : BusCreator  Inputs=11
  Bus Creator{8,10,13,15..17,24..25} (8 alike) : BusCreator  Inputs=2
  Bus Creator{5,19,21,23} (4 alike) : BusCreator  Inputs=4
  Read CAN Message10 : SF_CanService_Libs/Read CAN Message  typeCAN=Connected  channel=CAN_D  mEn=off  msgInfo=AMK_VCU_CAN_TorqueMode_factor_edited  msgItermStore=MCU3_287  msgIterm=MCU3_287  valid=on  stale=on  motoBit=off  setSignalName=on  flgCustomMonitorVariableRules=on  defineSignalName=off  prefixSignal='rx'  flgValTest=off  flgNoFixed=on  tSample=Task_Inherit  modeCode=Parameterless
  Read CAN Message11 : SF_CanService_Libs/Read CAN Message  typeCAN=Connected  channel=CAN_D  mEn=off  msgInfo=AMK_VCU_CAN_TorqueMode_factor_edited  msgItermStore=MCU3_289  msgIterm=MCU3_289  valid=on  stale=on  motoBit=off  setSignalName=on  flgCustomMonitorVariableRules=on  defineSignalName=off  prefixSignal='rx'  flgValTest=off  flgNoFixed=on  tSample=Task_Inherit  modeCode=Parameterless
  Read CAN Message12 : SF_CanService_Libs/Read CAN Message  typeCAN=Connected  channel=CAN_D  mEn=off  msgInfo=AMK_VCU_CAN_TorqueMode_factor_edited  msgItermStore=MCU4_288  msgIterm=MCU4_288  valid=on  stale=on  motoBit=off  setSignalName=on  flgCustomMonitorVariableRules=on  defineSignalName=off  prefixSignal='rx'  flgValTest=off  flgNoFixed=on  tSample=Task_Inherit  modeCode=Parameterless
  Read CAN Message13 : SF_CanService_Libs/Read CAN Message  typeCAN=Connected  channel=CAN_D  mEn=off  msgInfo=AMK_VCU_CAN_TorqueMode_factor_edited  msgItermStore=MCU4_28A  msgIterm=MCU4_28A  valid=on  stale=on  motoBit=off  setSignalName=on  flgCustomMonitorVariableRules=on  defineSignalName=off  prefixSignal='rx'  flgValTest=off  flgNoFixed=on  tSample=Task_Inherit  modeCode=Parameterless
  Read CAN Message2 : SF_CanService_Libs/Read CAN Message  typeCAN=Connected  channel=CAN_C  mEn=off  msgInfo=AMK_VCU_CAN_TorqueMode_factor_edited  msgItermStore=MCU1_283  msgIterm=MCU1_283  valid=on  stale=on  motoBit=off  setSignalName=on  flgCustomMonitorVariableRules=on  defineSignalName=off  prefixSignal='rx'  flgValTest=off  flgNoFixed=on  tSample=Task_Inherit  modeCode=Parameterless
  Read CAN Message5 : SF_CanService_Libs/Read CAN Message  typeCAN=Connected  channel=CAN_C  mEn=off  msgInfo=AMK_VCU_CAN_TorqueMode_factor_edited  msgItermStore=MCU1_285  msgIterm=MCU1_285  valid=on  stale=on  motoBit=off  setSignalName=on  flgCustomMonitorVariableRules=on  defineSignalName=off  prefixSignal='rx'  flgValTest=off  flgNoFixed=on  tSample=Task_Inherit  modeCode=Parameterless
  Read CAN Message6 : SF_CanService_Libs/Read CAN Message  typeCAN=Connected  channel=CAN_C  mEn=off  msgInfo=AMK_VCU_CAN_TorqueMode_factor_edited  msgItermStore=MCU2_284  msgIterm=MCU2_284  valid=on  stale=on  motoBit=off  setSignalName=on  flgCustomMonitorVariableRules=on  defineSignalName=off  prefixSignal='rx'  flgValTest=off  flgNoFixed=on  tSample=Task_Inherit  modeCode=Parameterless
  Read CAN Message9 : SF_CanService_Libs/Read CAN Message  typeCAN=Connected  channel=CAN_C  mEn=off  msgInfo=AMK_VCU_CAN_TorqueMode_factor_edited  msgItermStore=MCU2_286  msgIterm=MCU2_286  valid=on  stale=on  motoBit=off  setSignalName=on  flgCustomMonitorVariableRules=on  defineSignalName=off  prefixSignal='rx'  flgValTest=off  flgNoFixed=on  tSample=Task_Inherit  modeCode=Parameterless
  Terminator{7..14} (8 alike) : Terminator
  tag scope: Motor1_Tag1=global, Motor1_Tag2=global, Motor2_Tag1=global, Motor2_Tag2=global, Motor3_Tag1=global, Motor3_Tag2=global, Motor4_Tag1=global, Motor4_Tag2=global
  wires:
  Read CAN Message9/4 -> Bus Creator19/2  "rxMCU_TempIGBT"
  Read CAN Message9/1 -> Bus Creator16/1
  Bus Creator17/1 -> Terminator14/1
  Read CAN Message5/2 -> Bus Creator17/2
  Read CAN Message5/1 -> Bus Creator17/1
  Bus Creator19/1 -> [Motor2_Tag2]
  Read CAN Message11/2 -> Bus Creator15/2
  Read CAN Message12/1 -> Bus Creator8/1
  Read CAN Message2/1 -> Bus Creator24/1
  Bus Creator15/1 -> Terminator12/1
  Read CAN Message6/3 -> Bus Creator18/1  "rxMCU_TorqueCurrent"
  Read CAN Message12/3 -> Bus Creator22/1  "rxMCU_TorqueCurrent"
  Bus Creator16/1 -> Terminator13/1
  Bus Creator23/1 -> [Motor4_Tag2]
  Read CAN Message9/2 -> Bus Creator16/2
  Read CAN Message2/7 -> Bus Creator/5  "rxMCU_QuitInverterOn"
  Bus Creator/1 -> [Motor1_Tag1]
  Read CAN Message10/3 -> Bus Creator20/1  "rxMCU_TorqueCurrent"
  Bus Creator25/1 -> Terminator8/1
  Read CAN Message13/1 -> Bus Creator13/1
  Read CAN Message6/2 -> Bus Creator25/2
  Read CAN Message2/10 -> Bus Creator/8  "rxMCU_InverterOn"
  Bus Creator13/1 -> Terminator11/1
  Bus Creator10/1 -> Terminator9/1
  Read CAN Message6/10 -> Bus Creator18/8  "rxMCU_InverterOn"
  Read CAN Message11/1 -> Bus Creator15/1
  Read CAN Message13/3 -> Bus Creator23/1  "rxMCU_ErrorInfo"
  Read CAN Message10/2 -> Bus Creator10/2
  Read CAN Message12/2 -> Bus Creator8/2
  Bus Creator8/1 -> Terminator10/1
  Read CAN Message11/4 -> Bus Creator21/2  "rxMCU_TempIGBT"
  Read CAN Message5/3 -> Bus Creator5/1  "rxMCU_ErrorInfo"
  Read CAN Message6/12 -> Bus Creator18/10  "rxMCU_Warning"
  Read CAN Message10/7 -> Bus Creator20/5  "rxMCU_QuitInverterOn"
  Bus Creator24/1 -> Terminator7/1
  Read CAN Message2/2 -> Bus Creator24/2
  Bus Creator22/1 -> [Motor4_Tag1]
  Read CAN Message12/6 -> Bus Creator22/4  "rxMCU_DcOn"
  Read CAN Message10/11 -> Bus Creator20/9  "rxMCU_SystemReady"
  Read CAN Message2/8 -> Bus Creator/6  "rxMCU_Error"
  Read CAN Message5/4 -> Bus Creator5/2  "rxMCU_TempIGBT"
  Read CAN Message2/6 -> Bus Creator/4  "rxMCU_DcOn"
  Read CAN Message12/10 -> Bus Creator22/8  "rxMCU_InverterOn"
  Read CAN Message2/9 -> Bus Creator/7  "rxMCU_QuitDcOn"
  Read CAN Message2/3 -> Bus Creator/1  "rxMCU_TorqueCurrent"
  Read CAN Message6/8 -> Bus Creator18/6  "rxMCU_Error"
  Read CAN Message13/2 -> Bus Creator13/2
  Read CAN Message2/11 -> Bus Creator/9  "rxMCU_SystemReady"
  Bus Creator18/1 -> [Motor2_Tag1]
  Read CAN Message12/8 -> Bus Creator22/6  "rxMCU_Error"
  Read CAN Message6/5 -> Bus Creator18/3  "rxMCU_ActualVelocity"
  Read CAN Message12/4 -> Bus Creator22/2  "rxMCU_ActualTorque"
  Read CAN Message10/13 -> Bus Creator20/11  "rxMCU_Derating"
  Read CAN Message10/12 -> Bus Creator20/10  "rxMCU_Warning"
  Read CAN Message12/13 -> Bus Creator22/11  "rxMCU_Derating"
  Read CAN Message6/7 -> Bus Creator18/5  "rxMCU_QuitInverterOn"
  Read CAN Message6/13 -> Bus Creator18/11  "rxMCU_Derating"
  Read CAN Message10/4 -> Bus Creator20/2  "rxMCU_ActualTorque"
  Read CAN Message10/6 -> Bus Creator20/4  "rxMCU_DcOn"
  Read CAN Message10/10 -> Bus Creator20/8  "rxMCU_InverterOn"
  Read CAN Message10/9 -> Bus Creator20/7  "rxMCU_QuitDcOn"
  Read CAN Message12/12 -> Bus Creator22/10  "rxMCU_Warning"
  Read CAN Message12/7 -> Bus Creator22/5  "rxMCU_QuitInverterOn"
  Read CAN Message10/1 -> Bus Creator10/1
  Read CAN Message10/5 -> Bus Creator20/3  "rxMCU_ActualVelocity"
  Read CAN Message11/5 -> Bus Creator21/3  "rxMCU_TempInverter"
  Bus Creator5/1 -> [Motor1_Tag2]
  Bus Creator20/1 -> [Motor3_Tag1]
  Read CAN Message12/5 -> Bus Creator22/3  "rxMCU_ActualVelocity"
  Read CAN Message6/11 -> Bus Creator18/9  "rxMCU_SystemReady"
  Read CAN Message6/9 -> Bus Creator18/7  "rxMCU_QuitDcOn"
  Read CAN Message6/6 -> Bus Creator18/4  "rxMCU_DcOn"
  Bus Creator21/1 -> [Motor3_Tag2]
  Read CAN Message12/9 -> Bus Creator22/7  "rxMCU_QuitDcOn"
  Read CAN Message10/8 -> Bus Creator20/6  "rxMCU_Error"
  Read CAN Message13/4 -> Bus Creator23/2  "rxMCU_TempIGBT"
  Read CAN Message11/3 -> Bus Creator21/1  "rxMCU_ErrorInfo"
  Read CAN Message2/13 -> Bus Creator/11  "rxMCU_Derating"
  Read CAN Message9/3 -> Bus Creator19/1  "rxMCU_ErrorInfo"
  Read CAN Message2/12 -> Bus Creator/10  "rxMCU_Warning"
  Read CAN Message12/11 -> Bus Creator22/9  "rxMCU_SystemReady"
  Read CAN Message13/5 -> Bus Creator23/3  "rxMCU_TempInverter"
  Read CAN Message9/5 -> Bus Creator19/3  "rxMCU_TempInverter"
  Read CAN Message5/5 -> Bus Creator5/3  "rxMCU_TempInverter"
  Read CAN Message2/4 -> Bus Creator/2  "rxMCU_ActualTorque"
  Read CAN Message6/4 -> Bus Creator18/2  "rxMCU_ActualTorque"
  Read CAN Message2/5 -> Bus Creator/3  "rxMCU_ActualVelocity"
  Read CAN Message6/1 -> Bus Creator25/1
  Read CAN Message5/6 -> Bus Creator5/4  "rxMCU_TempMotor"
  Read CAN Message9/6 -> Bus Creator19/4  "rxMCU_TempMotor"
  Read CAN Message11/6 -> Bus Creator21/4  "rxMCU_TempMotor"
  Read CAN Message13/6 -> Bus Creator23/4  "rxMCU_TempMotor"
